simulink model "Integration"  (R2021a)
settings: Solver=VariableStepAuto  StartTime=0.0  StopTime=100  RelTol=1e-3
values from neighbouring files (symbols this model uses):
  data_map = [0 0 0 0 0 0 -0.696746291355 -1.00357651163 -1.30204806704 -1.55220205727 -1.77446676777 -2.12268177674 ... (7500 elements, 50x50x3)]    [TerrainData.mat]    (also in TerrainGenerator.m = zeros(terrain_x_indices, terrain_y_indices, 3))
  init_parameters = struct    [TerrainGenerator.m]    (also in WorkspaceLoader.m = load('init_parameters'))
libraries: vrlib x12
settings Model: Creator=16109  LastModifiedBy=16109

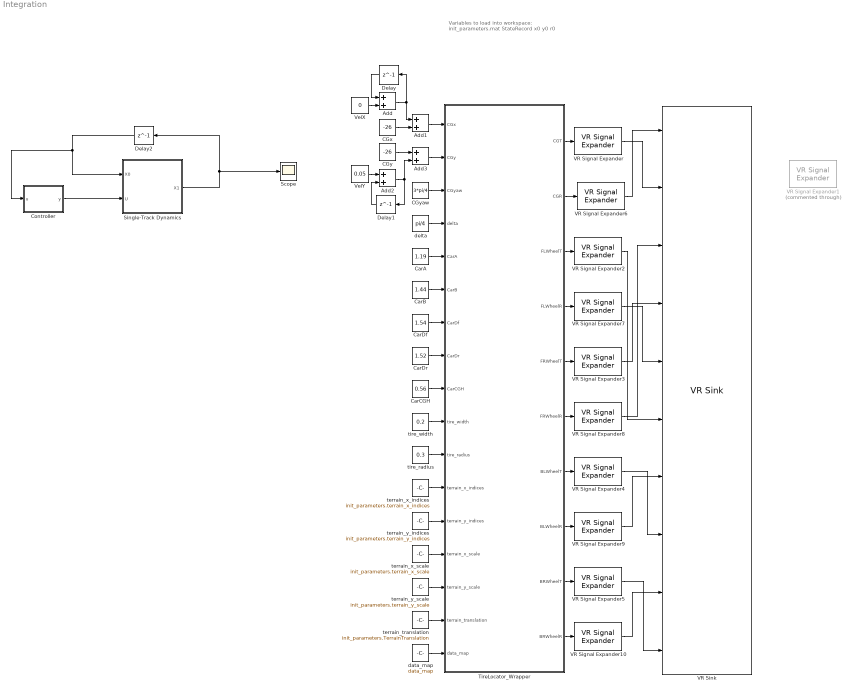
== system Integration ==
  note: Variables to load into workspace:
      | init_parameters.mat
      | StateRecord
      | x0
      | y0
      | r0
  Add{,1..3} (4 alike) : Sum
  CGx : Constant  Value=-26
  CGy : Constant  Value=-26
  CGyaw : Constant  Value=3*pi/4
  CarA : Constant  Value=1.19
  CarB : Constant  Value=1.44
  CarCGH : Constant  Value=0.56
  CarDf : Constant  Value=1.54
  CarDr : Constant  Value=1.52
  Controller : MATLAB Function  TreatAsAtomicUnit=on
  Delay : Delay  DelayLength=1
  Delay1 : Delay  DelayLength=1
  Delay2 : Delay  DelayLength=1  InitialCondition=[0 0 0 0 0 0 0 0]
  Scope : Scope
  Single-Track Dynamics : MATLAB Function  TreatAsAtomicUnit=on
  TireLocator_Wrapper : MATLAB Function  TreatAsAtomicUnit=on
  VR Signal Expander{,2..5} (5 alike) : vrlib/VR Signal Expander  outwidth=3  outidx=[1 3 2]
  VR Signal Expander1 : vrlib/VR Signal Expander  Commented=through  outwidth=3  outidx=[1]
  VR Signal Expander{6..10} (5 alike) : vrlib/VR Signal Expander  outwidth=4  outidx=[1 3 2 4]
  VR Sink : vrlib/VR Sink  InstantiateOnLoad=on  SampleTime=0.1  ViewEnable=on  RemoteChange=off  RemoteView=off  FieldsWritten=CarBody.rotation.4.1.1.double#CarBody.translation.3.1.1.double#FRWheel.rotation.4.1.1.double#FRWheel.translation.3.1.1.double#FLWheel.rotation.4.1.1.double#FLWheel.translation.3.1.1.double#BLWheel.rotation.4.1.1.double#BLWheel.translation.3.1.1.double#BRWheel.rotation.4.1.1.double#BRWheel.translation.3.1.1.double  WorldFileName=TerrainSimulation.x3d  AutoView=off  VideoDimensions=[]  AllowVariableSize=off
  VelX : Constant  Value=0
  VelY : Constant  Value=0.05
  data_map : Constant  Value=data_map  VectorParams1D=off
  delta : Constant  Value=pi/4
  terrain_translation : Constant  Value=init_parameters.TerrainTranslation
  terrain_x_indices : Constant  Value=init_parameters.terrain_x_indices
  terrain_x_scale : Constant  Value=init_parameters.terrain_x_scale
  terrain_y_indices : Constant  Value=init_parameters.terrain_y_indices
  terrain_y_scale : Constant  Value=init_parameters.terrain_y_scale
  tire_radius : Constant  Value=0.3
  tire_width : Constant  Value=0.2
  wires:
  TireLocator_Wrapper/1(CGT) -> VR Signal Expander/1
  VR Signal Expander/1 -> VR Sink/2
  TireLocator_Wrapper/2(CGR) -> VR Signal Expander6/1
  TireLocator_Wrapper/3(FLWheelT) -> VR Signal Expander2/1
  TireLocator_Wrapper/5(FRWheelT) -> VR Signal Expander3/1
  VR Signal Expander2/1 -> VR Sink/6
  VR Signal Expander3/1 -> VR Sink/4
  TireLocator_Wrapper/4(FLWheelR) -> VR Signal Expander7/1
  TireLocator_Wrapper/6(FRWheelR) -> VR Signal Expander8/1
  TireLocator_Wrapper/7(BLWheelT) -> VR Signal Expander4/1
  VR Signal Expander4/1 -> VR Sink/8
  TireLocator_Wrapper/9(BRWheelT) -> VR Signal Expander5/1
  VR Signal Expander5/1 -> VR Sink/10
  TireLocator_Wrapper/8(BLWheelR) -> VR Signal Expander9/1
  CGx/1 -> Add1/2
  CGy/1 -> Add3/1
  CGyaw/1 -> TireLocator_Wrapper/3(CGyaw)
  delta/1 -> TireLocator_Wrapper/4(delta)
  CarA/1 -> TireLocator_Wrapper/5(CarA)
  CarB/1 -> TireLocator_Wrapper/6(CarB)
  CarDf/1 -> TireLocator_Wrapper/7(CarDf)
  CarDr/1 -> TireLocator_Wrapper/8(CarDr)
  CarCGH/1 -> TireLocator_Wrapper/9(CarCGH)
  tire_width/1 -> TireLocator_Wrapper/10(tire_width)
  tire_radius/1 -> TireLocator_Wrapper/11(tire_radius)
  terrain_x_indices/1 -> TireLocator_Wrapper/12(terrain_x_indices)
  terrain_y_indices/1 -> TireLocator_Wrapper/13(terrain_y_indices)
  terrain_x_scale/1 -> TireLocator_Wrapper/14(terrain_x_scale)
  terrain_y_scale/1 -> TireLocator_Wrapper/15(terrain_y_scale)
  terrain_translation/1 -> TireLocator_Wrapper/16(terrain_translation)
  data_map/1 -> TireLocator_Wrapper/17(data_map)
  VR Signal Expander6/1 -> VR Sink/1
  VR Signal Expander7/1 -> VR Sink/5
  VR Signal Expander8/1 -> VR Sink/3
  VR Signal Expander9/1 -> VR Sink/7
  TireLocator_Wrapper/10(BRWheelR) -> VR Signal Expander10/1
  VelX/1 -> Add/2
  Add/1 -> Delay/1, Add1/1
  Delay/1 -> Add/1
  Add1/1 -> TireLocator_Wrapper/1(CGx)
  Add3/1 -> TireLocator_Wrapper/2(CGy)
  Add2/1 -> Add3/2, Delay1/1
  VelY/1 -> Add2/1
  Delay1/1 -> Add2/2
  VR Signal Expander10/1 -> VR Sink/9
  Single-Track Dynamics/1(X1) -> Delay2/1, Scope/1
  Delay2/1 -> Single-Track Dynamics/1(X0), Controller/1(u)
  Controller/1(y) -> Single-Track Dynamics/2(U)

== matlab function Integration/Controller ==
  data: u input; y output
function y = fcn(u)

y = [0 100 0];

== matlab function Integration/TireLocator_Wrapper ==
  data: CGT output; CGR output; CGx input; FLWheelT output; CGy input; CGyaw input; delta input; CarA input; CarB input; CarDf input; CarDr input; CarCGH input; tire_width input; tire_radius input; FLWheelR output; FRWheelT output; FRWheelR output; BLWheelT output; BLWheelR output; BRWheelT output; BRWheelR output; terrain_x_indices input; terrain_y_indices input; terrain_x_scale input; terrain_y_scale input; terrain_translation input; data_map input
function [CGT, CGR, FLWheelT, FLWheelR, FRWheelT, FRWheelR, BLWheelT, BLWheelR, BRWheelT, BRWheelR] = TireLocator_Wrapper(CGx, CGy, CGyaw, delta, CarA, CarB, CarDf, CarDr, CarCGH, tire_width, tire_radius, terrain_x_indices, terrain_y_indices, terrain_x_scale, terrain_y_scale, terrain_translation, data_map)
[CGT, CGR, FLWheelT, FLWheelR, FRWheelT, FRWheelR, BLWheelT, BLWheelR, BRWheelT, BRWheelR] = TireLocator(CGx, CGy, CGyaw, delta, CarA, CarB, CarDf, CarDr, CarCGH, tire_width, tire_radius, terrain_x_indices, terrain_y_indices, terrain_x_scale, terrain_y_scale, terrain_translation, data_map);
end

== matlab function Integration/Single-Track Dynamics ==
  data: X0 input; X1 output; U input
function X1 = Dynamics_wrapper(X0, U)
X1 = DynamicStepper(X0, U);
end
